simulink model "simulink"  (R2024b)
settings: Solver=ode4  StartTime=0.0  StopTime=10  FixedStep=Ts  RelTol=1e-3
values from neighbouring files (symbols this model uses):
  A = 0.5    [Parameteri_mport.m]
  alpha1_val = [10; 10; 10; 5; 5; 5]    [Parameteri_mport.m]
  alpha2_val = [5;   5;  5; 2; 2; 2]    [Parameteri_mport.m]
  delta = 0.05    [Parameteri_mport.m]
  dq0 = zeros(6,1)    [Parameteri_mport.m]
  epsilon = 0.01*ones(6,1)    [Parameteri_mport.m]
  eta1 = [20; 20; 20; 10; 10; 10]    [Parameteri_mport.m]
  eta2 = [10; 10; 10;  5;  5;  5]    [Parameteri_mport.m]
  gamma1 = [20; 20; 20; 20; 20; 20]    [Parameteri_mport.m]
  gamma1_val = 1.2    [Parameteri_mport.m]
  gamma2 = [0.2;   0.2;  0.2; 0.2;   0.2;  0.2]    [Parameteri_mport.m]
  gamma2_val = 0.8    [Parameteri_mport.m]
  k10 = [10; 10; 10;  5;  5;  5]    [Parameteri_mport.m]
  k20 = [5;  5;  5;  2; 2; 2]    [Parameteri_mport.m]
  k3 = [10; 10; 10;  5;  5;  5]    [Parameteri_mport.m]
  k4 = [5;  5;  5;  2; 2; 2]    [Parameteri_mport.m]
  lambda1 = [60; 60; 60; 50; 50; 50]    [Parameteri_mport.m]
  lambda2 = [6;   6;  6;  5;  5;  5]    [Parameteri_mport.m]
  omega_init = 1.0* ones(6,1)    [Parameteri_mport.m]
  phi_base = 0.02    [Parameteri_mport.m]
  phi_gain = 0.1    [Parameteri_mport.m]
  q0 = zeros(6,1)    [Parameteri_mport.m]
  tau_fall = 0.2 * ones(6,1)    [Parameteri_mport.m]
  tau_rise = 0.005 * ones(6,1)    [Parameteri_mport.m]
  Ts = 0.001    [Parameteri_mport.m]
  w = 1.0    (= 1)    [Parameteri_mport.m]
undefined symbols (not defined in the file or in its folder): beta1, beta2, beta3, omega_min
libraries: robotmaniplib x6, simulink x1
settings Model: Creator=35340  LastModifiedBy=35340
settings DataIOCC: SaveFormat=Array

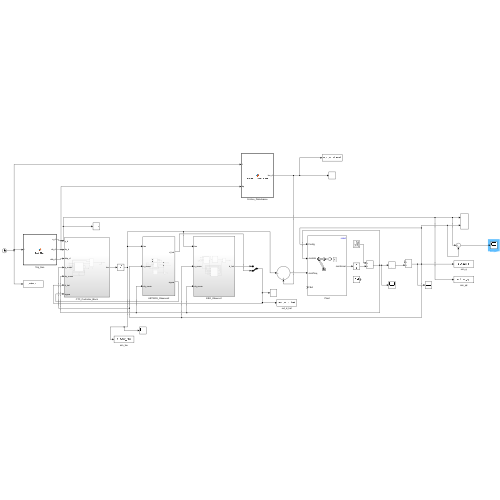
[thumbnail: Simulink's stored preview of the top-level diagram]
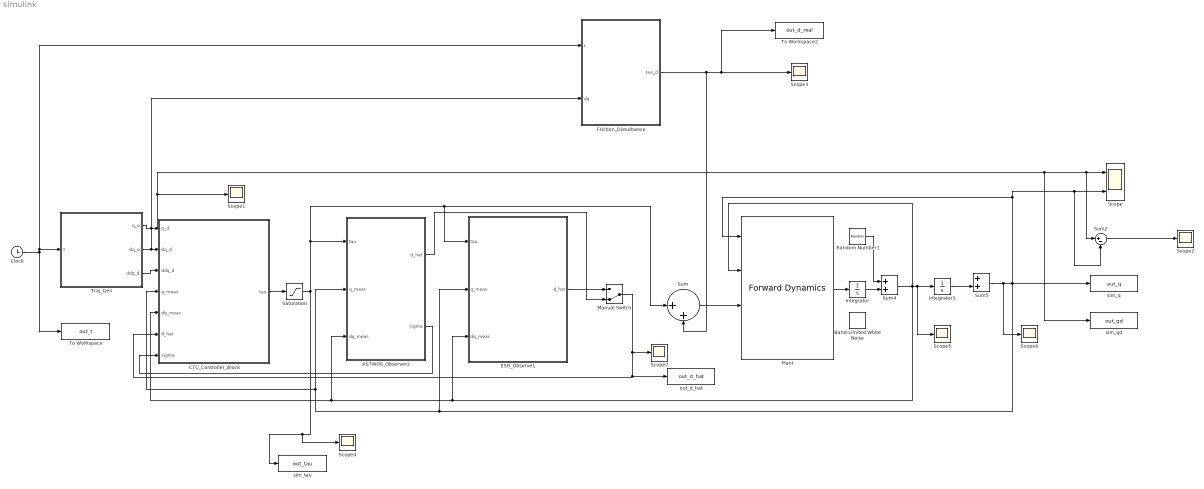
== system simulink ==
  ASTWOS_Observer2 : Subsystem
  Band-Limited White Noise : simulink/Sources/Band-Limited White Noise  Cov=1e-8  Ts=Ts  seed=[23341 34 123 543 233 1]
  CTC_Controller_Block : Subsystem
  Clock : Clock
  ESO_Observe1 : Subsystem
  Friction_Disturbance : MATLAB Function  TreatAsAtomicUnit=on
  Integrator : Integrator  InitialCondition=dq0
  Integrator1 : Integrator  InitialCondition=q0
  Manual Switch : ManualSwitch  CurrentSetting=0
  Plant : robotmaniplib/Forward Dynamics  RigidBodyTree=robot  SimulateUsing=Interpreted execution
  Random Number1 : RandomNumber  Variance=1e-6 * ones(6,1)  Seed=[1; 2; 3; 4; 5; 6]  SampleTime=Ts
  Saturation : Saturate  UpperLimit=150  LowerLimit=-150
  Scope : Scope  NumInputPorts=2
  Scope{1..7} (7 alike) : Scope
  Sum : Sum  Inputs=|++
  Sum2 : Sum  Inputs=|+-
  Sum4 : Sum
  Sum5 : Sum
  To Workspace : ToWorkspace  VariableName=out_t  SaveFormat=Timeseries  SampleTime=-1
  To Workspace2 : ToWorkspace  VariableName=out_d_real  SampleTime=-1
      settings: Save2DSignal=2-D array (concatenate along first dimension)
  Traj_Gen : MATLAB Function  TreatAsAtomicUnit=on
  out_d_hat : ToWorkspace  VariableName=out_d_hat  SampleTime=-1
  sim_q : ToWorkspace  VariableName=out_q  SampleTime=-1
  sim_qd : ToWorkspace  VariableName=out_qd  SampleTime=-1
  sim_tau : ToWorkspace  VariableName=out_tau  SampleTime=-1
  wires:
  Traj_Gen/3(ddq_d) -> CTC_Controller_Block/3(ddq_d)
  Traj_Gen/2(dq_d) -> Friction_Disturbance/2(dq), CTC_Controller_Block/2(dq_d)
  Plant/1 -> Integrator/1
  CTC_Controller_Block/1(tau) -> Saturation/1
  Manual Switch/1 -> Scope7/1, CTC_Controller_Block/6(d_hat), out_d_hat/1
  Sum/1 -> Plant/3
  Integrator/1 -> Sum4/2
  Integrator1/1 -> Sum5/2
  Sum4/1 -> Scope5/1, Integrator1/1, Plant/2, ESO_Observe1/3(dq_meas), ASTWOS_Observer2/3(dq_meas), CTC_Controller_Block/5(dq_meas)
  Traj_Gen/1(q_d) -> Scope1/1, sim_qd/1, Sum2/1, Scope/1, CTC_Controller_Block/1(q_d)
  Sum5/1 -> Scope6/1, Sum2/2, Scope/2, Plant/1, ESO_Observe1/2(q_meas), ASTWOS_Observer2/2(q_meas), CTC_Controller_Block/4(q_meas), sim_q/1
  ESO_Observe1/1(d_hat) -> Manual Switch/1
  Saturation/1 -> ASTWOS_Observer2/1(tau), ESO_Observe1/1(tau), Sum/1, Scope4/1, sim_tau/1
  Random Number1/1 -> Sum4/1
  Clock/1 -> Friction_Disturbance/1(t), Traj_Gen/1(t), To Workspace/1
  Friction_Disturbance/1(tau_d) -> Sum/2, To Workspace2/1, Scope3/1
  Sum2/1 -> Scope2/1
  ASTWOS_Observer2/1(d_hat) -> Manual Switch/2
  ASTWOS_Observer2/2(sigma) -> CTC_Controller_Block/7(sigma)

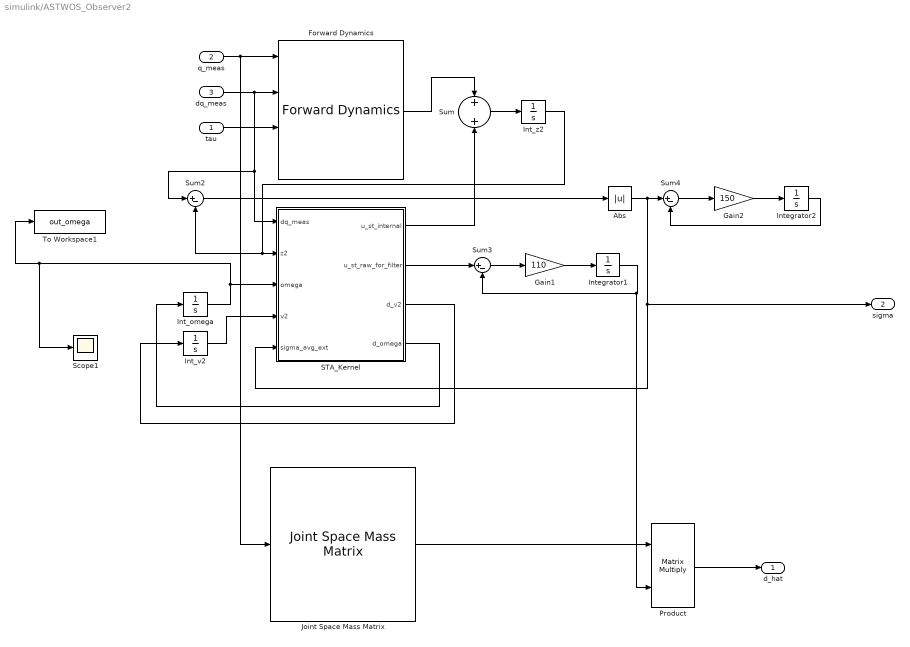
== system simulink/ASTWOS_Observer2 ==
  tau : Inport
  q_meas : Inport  Port=2
  dq_meas : Inport  Port=3
  Abs : Abs  SaturateOnIntegerOverflow=off
  Forward Dynamics : robotmaniplib/Forward Dynamics  RigidBodyTree=robot  SimulateUsing=Interpreted execution
  Gain1 : Gain  Gain=110
  Gain2 : Gain  Gain=150
  Int_omega : Integrator  InitialCondition=omega_init
  Int_v2 : Integrator  InitialCondition=zeros(6,1)
  Int_z2 : Integrator  InitialCondition=zeros(6,1)
  Integrator1 : Integrator  InitialCondition=zeros(6,1)
  Integrator2 : Integrator  InitialCondition=zeros(6,1)
  Joint Space Mass Matrix : robotmaniplib/Joint Space Mass Matrix  RigidBodyTree=robot  SimulateUsing=Interpreted execution
  Product : Product  Multiplication=Matrix(*)
  STA_Kernel : MATLAB Function  TreatAsAtomicUnit=on
  Scope1 : Scope
  Sum : Sum
  Sum2 : Sum  Inputs=|+-
  Sum3 : Sum  Inputs=|+-
  Sum4 : Sum  Inputs=|+-
  To Workspace1 : ToWorkspace  VariableName=out_omega  SampleTime=-1
      settings: Save2DSignal=2-D array (concatenate along first dimension)
  d_hat : Outport
  sigma : Outport  Port=2
  wires:
  q_meas/1 -> Forward Dynamics/1, Joint Space Mass Matrix/1
  dq_meas/1 -> STA_Kernel/1(dq_meas), Sum2/1, Forward Dynamics/2
  tau/1 -> Forward Dynamics/3
  Forward Dynamics/1 -> Sum/1
  Sum/1 -> Int_z2/1
  STA_Kernel/4(d_omega) -> Int_omega/1
  Int_omega/1 -> Scope1/1, To Workspace1/1, STA_Kernel/3(omega)
  Joint Space Mass Matrix/1 -> Product/1
  Int_v2/1 -> STA_Kernel/4(v2)
  STA_Kernel/1(u_st_internal) -> Sum/2
  STA_Kernel/3(d_v2) -> Int_v2/1
  Int_z2/1 -> STA_Kernel/2(z2), Sum2/2
  Product/1 -> d_hat/1
  STA_Kernel/2(u_st_raw_for_filter) -> Sum3/1
  Sum2/1 -> Abs/1
  Sum3/1 -> Gain1/1
  Gain1/1 -> Integrator1/1
  Sum4/1 -> Gain2/1
  Gain2/1 -> Integrator2/1
  Abs/1 -> STA_Kernel/5(sigma_avg_ext), sigma/1, Sum4/1
  Integrator1/1 -> Product/2, Sum3/2
  Integrator2/1 -> Sum4/2

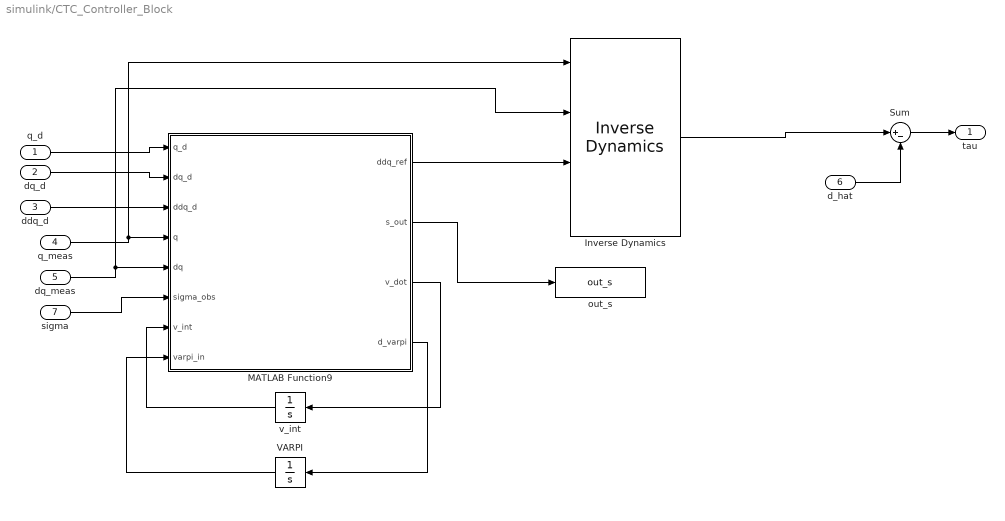
== system simulink/CTC_Controller_Block ==
  q_d : Inport
  dq_d : Inport  Port=2
  ddq_d : Inport  Port=3
  q_meas : Inport  Port=4
  dq_meas : Inport  Port=5
  d_hat : Inport  Port=6
  sigma : Inport  Port=7
  Inverse Dynamics : robotmaniplib/Inverse Dynamics  RigidBodyTree=robot  SimulateUsing=Interpreted execution
  MATLAB Function9 : MATLAB Function  TreatAsAtomicUnit=on
  Sum : Sum  Inputs=|+-
  VARPI : Integrator  InitialCondition=zeros(6,1)
  out_s : ToWorkspace  VariableName=out_s  SampleTime=-1
  v_int : Integrator  InitialCondition=zeros(6,1)
  tau : Outport
  wires:
  ddq_d/1 -> MATLAB Function9/3(ddq_d)
  q_meas/1 -> Inverse Dynamics/1, MATLAB Function9/4(q)
  dq_meas/1 -> Inverse Dynamics/2, MATLAB Function9/5(dq)
  Inverse Dynamics/1 -> Sum/1
  Sum/1 -> tau/1
  q_d/1 -> MATLAB Function9/1(q_d)
  dq_d/1 -> MATLAB Function9/2(dq_d)
  d_hat/1 -> Sum/2
  MATLAB Function9/1(ddq_ref) -> Inverse Dynamics/3
  MATLAB Function9/2(s_out) -> out_s/1
  v_int/1 -> MATLAB Function9/7(v_int)
  MATLAB Function9/3(v_dot) -> v_int/1
  sigma/1 -> MATLAB Function9/6(sigma_obs)
  MATLAB Function9/4(d_varpi) -> VARPI/1
  VARPI/1 -> MATLAB Function9/8(varpi_in)

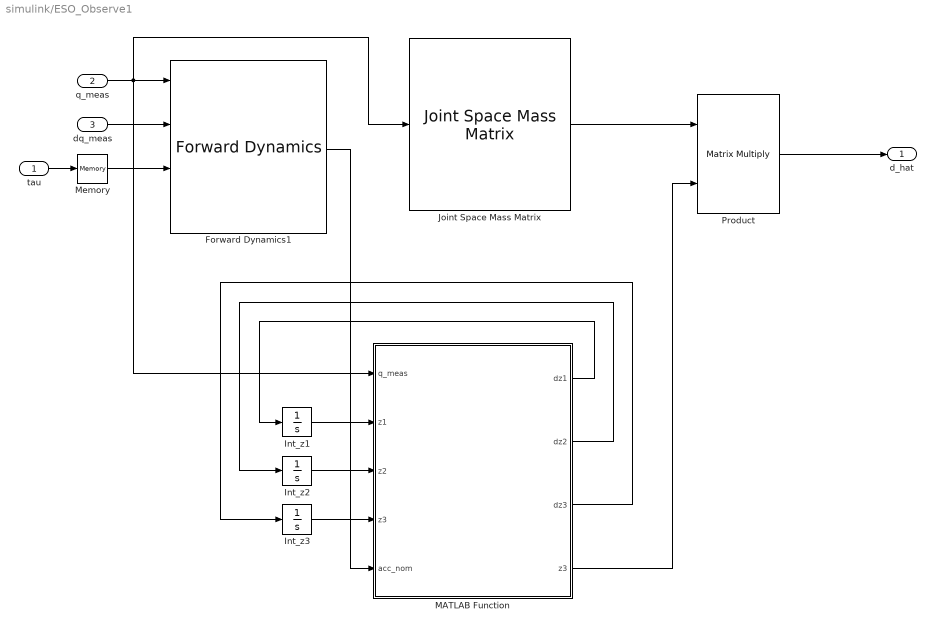
== system simulink/ESO_Observe1 ==
  tau : Inport
  q_meas : Inport  Port=2
  dq_meas : Inport  Port=3
  Forward Dynamics1 : robotmaniplib/Forward Dynamics  RigidBodyTree=robot  SimulateUsing=Interpreted execution
  Int_z1 : Integrator  InitialCondition=q0
  Int_z2 : Integrator  InitialCondition=dq0
  Int_z3 : Integrator  InitialCondition=zeros(6,1)
  Joint Space Mass Matrix : robotmaniplib/Joint Space Mass Matrix  RigidBodyTree=robot  SimulateUsing=Interpreted execution
  MATLAB Function : MATLAB Function  TreatAsAtomicUnit=on
  Memory : Memory  InitialCondition=zeros(6,1)
  Product : Product  Multiplication=Matrix(*)
  d_hat : Outport
  wires:
  dq_meas/1 -> Forward Dynamics1/2
  q_meas/1 -> MATLAB Function/1(q_meas), Joint Space Mass Matrix/1, Forward Dynamics1/1
  tau/1 -> Memory/1
  Int_z1/1 -> MATLAB Function/2(z1)
  Int_z2/1 -> MATLAB Function/3(z2)
  Int_z3/1 -> MATLAB Function/4("z3 ")
  MATLAB Function/1(dz1) -> Int_z1/1
  MATLAB Function/2(dz2) -> Int_z2/1
  MATLAB Function/3(dz3) -> Int_z3/1
  Product/1 -> d_hat/1
  Joint Space Mass Matrix/1 -> Product/1
  MATLAB Function/4(z3) -> Product/2
  Forward Dynamics1/1 -> MATLAB Function/5(acc_nom)
  Memory/1 -> Forward Dynamics1/3

== matlab function simulink/ASTWOS_Observer2/STA_Kernel ==
  data: dq_meas input; u_st_internal output; u_st_raw_for_filter output; z2 input; omega input; v2 input; sigma_avg_ext input; lambda1 parameter; lambda2 parameter; gamma1 parameter; epsilon parameter; omega_min parameter; delta parameter; gamma2 parameter; d_v2 output; d_omega output
function [u_st_internal, u_st_raw_for_filter, d_v2, d_omega] = ASTWOS_Kernel(dq_meas, z2, omega, v2, sigma_avg_ext, lambda1, lambda2, gamma1, epsilon, omega_min, delta, gamma2)
    % =========================================================
    % 纯净版 ASTWOS 核心：移除所有 persistent 变量
    % 将滤波操作转移到 Simulink 外部标准模块完成
    % =========================================================
    
    % 1. 计算瞬时速度误差
    sigma = dq_meas - z2;
    
    % 2. 平滑符号函数
    sig_sigma = tanh(sigma ./ delta);
    omega_max = 30.0; 
    
    % 3. 自适应律 (现在依赖外部传进来的平滑误差 sigma_avg_ext)
    d_omega = zeros(6,1);
    hyst_factor = 1.1;
    for i=1:6
        eps_low = epsilon(i);
        eps_high = epsilon(i) * hyst_factor;
        
        % 使用外部传进来的平均值进行判断
        metric = sigma_avg_ext(i); 
        
        if metric > eps_high
            if omega(i) < omega_max
                d_omega(i) = gamma1(i);
            else
                d_omega(i) = 0;
            end
        elseif metric < eps_low
            if omega(i) > omega_min(i)
                d_omega(i) = -gamma2(i) * omega(i);
            else
                d_omega(i) = 0;
            end
        else
            d_omega(i) = 0;
        end
    end
    
    % 4. 计算注入项
    k1 = lambda1 .* sqrt(omega);
    k2 = lambda2 .* omega;
    
    v1 = k1 .* sqrt(abs(sigma)) .* sig_sigma;
    d_v2 = k2 .* sig_sigma;
    
    % 5. 原始总注入项
    u_st_raw = v1 + v2; 
    
    % 6. 端口输出分配
    % 给内部积分器算 z2 用 (无滤波，保持敏感)
    u_st_internal = u_st_raw; 
    
    % 给外部滤波器用 (用来算平滑的 d_hat)
    u_st_raw_for_filter = u_st_raw; 



end

== matlab function simulink/Traj_Gen ==
  data: t input; q_d output; dq_d output; ddq_d output; A parameter; w parameter; q0 parameter
function [q_d, dq_d, ddq_d] = Traj_Gen(t, A, w, q0)
    % 升级版：5阶傅里叶级数拟合三角波 (视觉更尖锐，数学依然安全)
    q_d = zeros(6,1);
    dq_d = zeros(6,1);
    ddq_d = zeros(6,1);
    
    for i = 1:3
        % 位置
        q_d(i) = q0(i) + A * (sin(w*t) - (1/9)*sin(3*w*t) + (1/25)*sin(5*w*t) - (1/49)*sin(7*w*t) + (1/81)*sin(9*w*t));
        % 速度
        dq_d(i) = A * w * (cos(w*t) - (1/3)*cos(3*w*t) + (1/5)*cos(5*w*t) - (1/7)*cos(7*w*t) + (1/9)*cos(9*w*t));
        % 加速度
        ddq_d(i) = -A * w^2 * (sin(w*t) - sin(3*w*t) + sin(5*w*t) - sin(7*w*t) + sin(9*w*t));
    end
    
    for i = 4:6
        q_d(i) = q0(i);
    end
end

== matlab function simulink/Friction_Disturbance ==
  data: t input; tau_d output; dq input
function tau_d = Friction_Disturbance(t, dq)
    % =========================================================
    % 模拟真实机械臂复合扰动 (周期震荡 + 库仑摩擦)
    % 输入:
    %   t : 仿真时间 (标量)
    %   dq: 关节实际速度 (6x1 向量)
    % 输出:
    %   tau_d: 扰动力矩 (6x1 向量)
    % =========================================================
    
    % 1. 初始化 6x1 零向量 (因为 UR5 有 6 个关节)
    tau_d = zeros(6, 1);
    
    % 2. 为了防止 Simulink 在速度为 0 时因 sign 函数产生代数环或步长报错，
    % 我们在工程上通常用极小宽度的 tanh 代替纯 sign 函数。
    % 效果完全一样，但数值计算极其稳定！
    vel_threshold = 0.05; 
    
    % 3. 严格按照论文公式写入前 3 个大臂关节的干扰
    % 关节 1
    tau_d(1) = 15 * sin(t) + 10 * tanh(dq(1) / vel_threshold);
    
    % 关节 2
    tau_d(2) = 10 * sin(t) + 10 * tanh(dq(2) / vel_threshold);
    
    % 关节 3
    tau_d(3) = 5 * sin(t) + 10 * tanh(dq(3) / vel_threshold);
    
    % 关节 4, 5, 6 保持为 0 (无需写代码，上面已经初始化为0了)
end

== matlab function simulink/ESO_Observe1/MATLAB Function ==
  data: q_meas input; dz1 output; z1 input; z2 input; z3 input; acc_nom input; dz2 output; dz3 output; z3 output; beta1 parameter; beta2 parameter; beta3 parameter
function [dz1, dz2, dz3, z3] = ESO_Kernel(q_meas, z1, z2, z3, acc_nom, beta1, beta2, beta3)
    % 1. 观测误差
    e = q_meas - z1;
    
    % 2. 状态导数 (Linear ESO)
    dz1 = z2 + beta1 .* e;
    dz2 = acc_nom + z3 + beta2 .* e;
    dz3 = beta3 .* e;
    
    % 输出 z3 给 d_hat 计算
end

== matlab function simulink/CTC_Controller_Block/MATLAB Function9 ==
  data: q_d input; ddq_ref output; dq_d input; ddq_d input; q input; dq input; sigma_obs input; v_int input; varpi_in input; alpha1_val parameter; alpha2_val parameter; gamma1_val parameter; s_out output; v_dot output; gamma2_val parameter; k10 parameter; k20 parameter; eta1 parameter; eta2 parameter; k3 parameter; k4 parameter; d_varpi output; tau_rise parameter; tau_fall parameter; phi_base parameter; phi_gain parameter
function [ddq_ref, s_out, v_dot, d_varpi] = ASTO_FxST_NTSMC_Controller(q_d, dq_d, ddq_d, q, dq, sigma_obs, v_int, varpi_in, alpha1_val, alpha2_val, gamma1_val, gamma2_val, k10, k20, eta1, eta2, k3, k4, tau_rise, tau_fall, phi_base, phi_gain)
    % =====================================================================
    % ASTO-FxST-NTSMC 终极完全体 (包含非对称滤波 + 动态边界层)
    % =====================================================================
    
    e = q_d - q;       
    de = dq_d - dq;    
    eps_e = 1e-4; 
    
    p = 1.5; 
    q_pow = 2.0; 
    
    ddq_ref = zeros(6,1);
    s = zeros(6,1);
    v_dot = zeros(6,1); 
    d_varpi = zeros(6,1); % 新增：联动因子的导数 (输出给外部积分)
    
    for i = 1:6
        % -------------------------------------------------------------
        % 创新 1：动态自适应边界层 (Dynamic Boundary Layer)
        % -------------------------------------------------------------
        abs_sig_obs = abs(sigma_obs(i));
        % 误差越大，边界层越宽(越平滑)；误差越小，边界层越窄(越精准)
        phi_s = phi_base + phi_gain * abs_sig_obs;
        
        % A. 滑模面
        term1_s = alpha1_val(i) * (abs(e(i))^gamma1_val) * sign(e(i));
        term2_s = alpha2_val(i) * (abs(e(i))^gamma2_val) * sign(e(i));
        s(i) = de(i) + term1_s + term2_s;
        
        % B. 等效控制微分项
        abs_e_safe = abs(e(i));
        if abs_e_safe < eps_e
            abs_e_safe = eps_e;
        end
        d_term1 = alpha1_val(i) * gamma1_val * (abs(e(i))^(gamma1_val - 1)) * de(i); 
        d_term2 = alpha2_val(i) * gamma2_val * (abs_e_safe^(gamma2_val - 1)) * de(i);
        
        % -------------------------------------------------------------
        % 创新 2：非对称连续滤波联动机制 (Asymmetric Continuous Linkage)
        % -------------------------------------------------------------
        eps_link = 0.03;  
        mu = 50;         
        
        % 1. 计算目标联动因子 (代数目标值)
        varpi_target = 1 / (1 + exp(-mu * (abs_sig_obs - eps_link)));
        
        % 2. 核心数学原理：非对称一阶微分方程
        % 让 Simulink 原生的 Integrator 去做积分，获得绝对平滑的 varpi_in
        if varpi_target > varpi_in(i)
            % 上升期：反应迅速，抗击扰动
            d_varpi(i) = (varpi_target - varpi_in(i)) / tau_rise(i);
        else
            % 下降期：衰减缓慢，防止抖振
            d_varpi(i) = (varpi_target - varpi_in(i)) / tau_fall(i);
        end
        
        % 3. 使用平滑后的状态变量 varpi_in 计算增益
        k1_t = k10(i) + eta1(i) * varpi_in(i);
        k2_t = k20(i) + eta2(i) * varpi_in(i);
        
        % -------------------------------------------------------------
        % C. FxST 趋近律 (使用动态边界层 phi_s)
        % -------------------------------------------------------------
        sig_s = tanh(s(i) / phi_s); 
        
        u_prop = k1_t * sqrt(abs(s(i))) * sig_s + k3(i) * (abs(s(i))^p) * sig_s;
        v_dot(i) = k2_t * sig_s + k4(i) * (abs(s(i))^q_pow) * sig_s;
        u_rob = u_prop + v_int(i);
                  
        % D. 合成最终参考加速度
        ddq_ref(i) = ddq_d(i) + d_term1 + d_term2 + u_rob;
        
        % 物理限幅
        limit_val = 200; 
        if ddq_ref(i) > limit_val
            ddq_ref(i) = limit_val;
        elseif ddq_ref(i) < -limit_val
            ddq_ref(i) = -limit_val;
        end
    end
    s_out = s;
end
